simulink model "Verifica_LMI"  (R2025b)
settings: Solver=VariableStepAuto  StartTime=0.0  StopTime=50.0  RelTol=1e-3
values from neighbouring files (symbols this model uses):
  A = double(subs(A_sym, [x; u], [x_star; u_star]))    [Main_20042026.m]
  B = double(subs(B_sym, [x; u], [x_star; u_star]))    [Main_20042026.m]
  C = double(subs(C_sym, [x; u], [x_star; u_star]))    [Main_20042026.m]
  D = double(subs(D_sym, [x; u], [x_star; u_star]))    [Main_20042026.m]
  h0 = [0.3 ... (first row only)    [Main_20042026.m]
  h_ref = [h1_ref_lmi ... (first row only)    [Main_20042026.m]
  K_LMI = -L/Q    [Main_20042026.m]
  N = pinv(gain)    [Main_20042026.m]
settings Model: Creator=salvo  LastModifiedBy=salvo

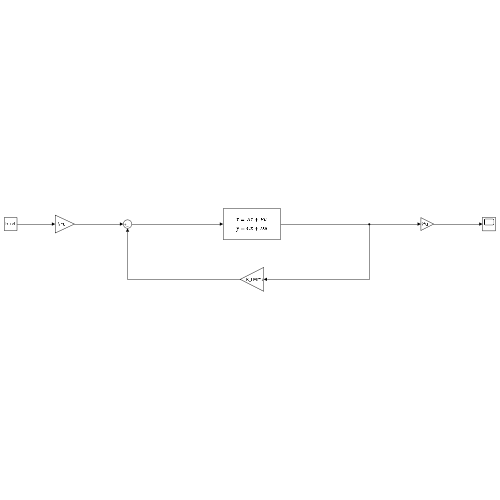
[thumbnail: Simulink's stored preview of the top-level diagram]
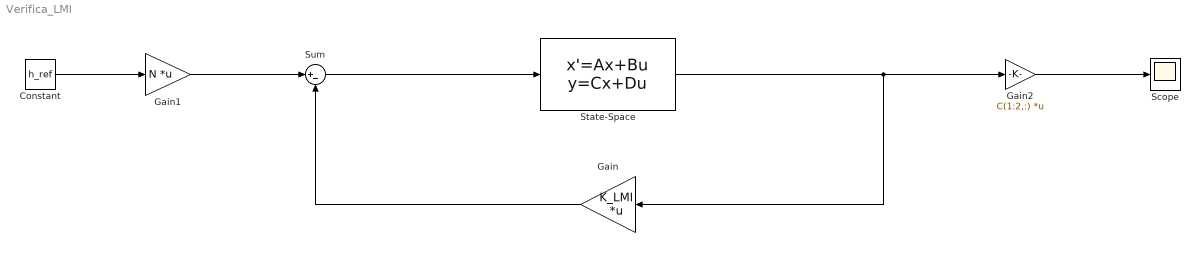
== system Verifica_LMI ==
  Constant : Constant  Value=h_ref
  Gain : Gain  Gain=K_LMI  Multiplication=Matrix(K*u)
  Gain1 : Gain  Gain=N  Multiplication=Matrix(K*u)
  Gain2 : Gain  Gain=C(1:2,:)  Multiplication=Matrix(K*u)
  Scope : Scope
      settings: ActiveDisplayYMinimum=-0.41289523795719629  ActiveDisplayYMaximum=1.4604805549767974
  State-Space : StateSpace  A=A  B=B  C=C  D=D  InitialCondition=h0
  Sum : Sum  Inputs=|+-
  wires:
  Sum/1 -> State-Space/1
  Gain1/1 -> Sum/1
  Constant/1 -> Gain1/1
  Gain/1 -> Sum/2
  State-Space/1 -> Gain2/1, Gain/1
  Gain2/1 -> Scope/1
